simulink model "pm4_motor"  (R2017a)
settings: Solver=VariableStepAuto  StartTime=0.0  StopTime=3.0  RelTol=1e-3
libraries: simulink x1
settings Model: Creator=robotica  LastModifiedBy=robotica

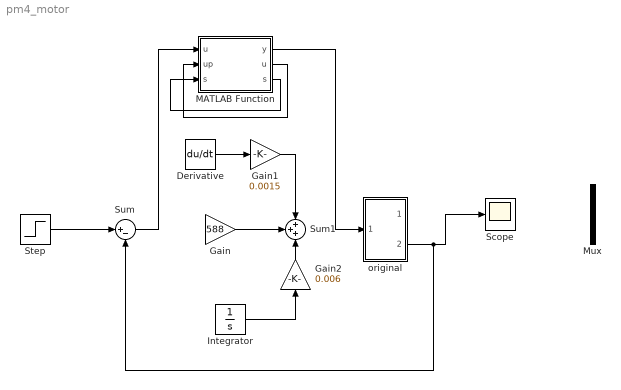
== system pm4_motor ==
  Derivative : Derivative
  Gain : Gain  Gain=588
  Gain1 : Gain  Gain=0.0015
  Gain2 : Gain  Gain=0.006
  Integrator : Integrator
  MATLAB Function : MATLAB Function  TreatAsAtomicUnit=on
  Mux : Mux  Inputs=2
  Scope : Scope
  Step : Step  SampleTime=1
  Sum : Sum  Inputs=|+-
  Sum1 : Sum  Inputs=+++
  original : Subsystem
  wires:
  Step/1 -> Sum/1
  Gain/1 -> Sum1/2
  Derivative/1 -> Gain1/1
  Gain1/1 -> Sum1/1
  Integrator/1 -> Gain2/1
  Gain2/1 -> Sum1/3
  original/2(clean) -> Sum/2, Scope/1
  Sum/1 -> MATLAB Function/1("u ")
  MATLAB Function/1(y) -> original/1(signal)
  MATLAB Function/2(u) -> MATLAB Function/2(up)
  MATLAB Function/3(s) -> MATLAB Function/3("s ")

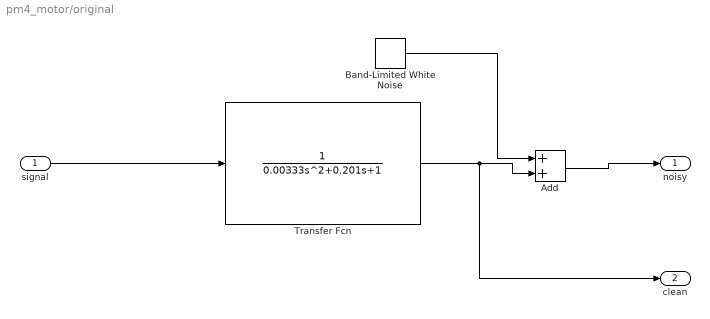
== system pm4_motor/original ==
  signal : Inport
  Add : Sum
  Band-Limited White Noise : simulink/Sources/Band-Limited White Noise  Cov=[0.0000001]  Ts=0.001  seed=[23341]
  Transfer Fcn : TransferFcn  Denominator=[0.00333 0.201 1]
  noisy : Outport
  clean : Outport  Port=2
  wires:
  Transfer Fcn/1 -> clean/1, Add/2
  Band-Limited White Noise/1 -> Add/1
  Add/1 -> noisy/1
  signal/1 -> Transfer Fcn/1

== matlab function pm4_motor/MATLAB Function ==
  data: u input; y output; up input; s input; u output; s output
function [y, u, s] = fcn(u, up  , s  )
kp = 40;
ki = 2;
kd = 10;
yp = u-up;
s = s + u;
y = ki*s+kd*yp+kp*u;
